simulink model "ExtraCredit_1"  (R2024a)
settings: Solver=VariableStepAuto  StartTime=0.0  StopTime=3500  MaxStep=.001  RelTol=1e-3
undefined symbols (not defined in the file): g, rh, y0
settings Model: Creator=gzipprich  LastModifiedBy=gzipprich

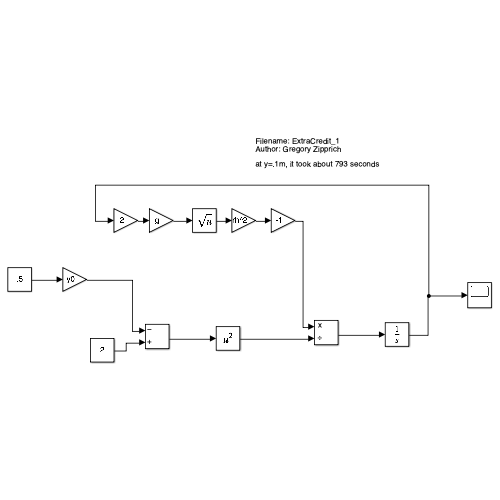
[thumbnail: Simulink's stored preview of the top-level diagram]
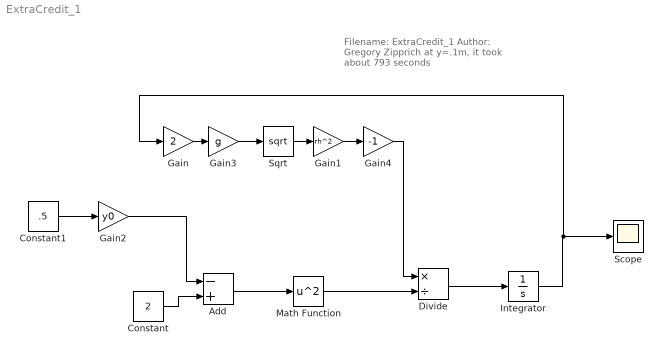
== system ExtraCredit_1 ==
  note: Filename: ExtraCredit_1
      | Author: Gregory Zipprich
      |
      | at y=.1m, it took about 793 seconds
  Add : Sum  Inputs=-+
  Constant : Constant  Value=2
  Constant1 : Constant  Value=.5
  Divide : Product  Inputs=*/
  Gain : Gain  Gain=2
  Gain1 : Gain  Gain=rh^2
  Gain2 : Gain  Gain=y0
  Gain3 : Gain  Gain=g
  Gain4 : Gain  Gain=-1
  Integrator : Integrator  InitialCondition=2
  Math Function : Math  Operator=square
  Scope : Scope
  Sqrt : Sqrt
  wires:
  Sqrt/1 -> Gain1/1
  Gain2/1 -> Add/1
  Constant/1 -> Add/2
  Add/1 -> Math Function/1
  Math Function/1 -> Divide/2
  Divide/1 -> Integrator/1
  Constant1/1 -> Gain2/1
  Gain1/1 -> Gain4/1
  Gain4/1 -> Divide/1
  Gain/1 -> Gain3/1
  Gain3/1 -> Sqrt/1
  Integrator/1 -> Gain/1, Scope/1
